simulink model "test8_sub_named_with_slash_orig"  (R2016b)
settings: Solver=VariableStepAuto  StartTime=0.0  StopTime=10.0  RelTol=1e-3
settings Model: Creator=gm  LastModifiedBy=gm

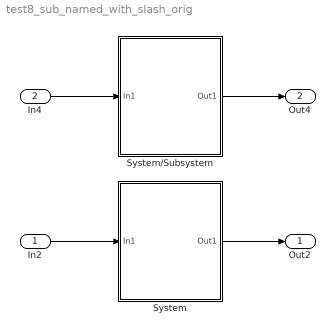
== system test8_sub_named_with_slash_orig ==
  In2 : Inport
  In4 : Inport  Port=2
  System : Subsystem
  System/Subsystem : Subsystem
  Out2 : Outport
  Out4 : Outport  Port=2
  wires:
  In2/1 -> System/1(In1)
  System/1(Out1) -> Out2/1
  In4/1 -> System/Subsystem/1(In1)
  System/Subsystem/1(Out1) -> Out4/1

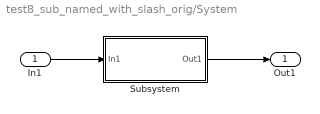
== system test8_sub_named_with_slash_orig/System ==
  In1 : Inport
  Subsystem : Subsystem
  Out1 : Outport
  wires:
  In1/1 -> Subsystem/1(In1)
  Subsystem/1(Out1) -> Out1/1

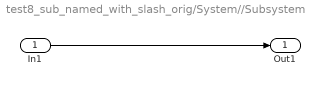
== system test8_sub_named_with_slash_orig/System//Subsystem ==
  In1 : Inport
  Out1 : Outport
  wires:
  In1/1 -> Out1/1

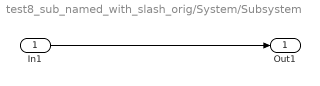
== system test8_sub_named_with_slash_orig/System/Subsystem ==
  In1 : Inport
  Out1 : Outport
  wires:
  In1/1 -> Out1/1
